simulink model "Csm_HighLvlArchitecture"  (R2017b)
settings: Solver=VariableStepAuto  StartTime=0.0  StopTime=10.0  RelTol=1e-3
undefined symbols (not defined in the file): accEgoVeh, Acceleration, apsEgoVeh, bpEgoVeh, Coasting, Control, CurrentDrivingLane, Curvature, CutIn, CutOut, Decelleration, distEgo2TS, distPredVeh, EgoVeh_State, EgoVehicle, GRG, Idle, ITS, Localization, Management, MATLAB, Mobileye, Obstacles, Obstacles_State, Perception, posEgoVeh, posGear, posTrafficSignal, PrecedingVehicle, Prediction, Python, Regen, Run, Slope, spdEgoVeh, spdMot, spdPredVeh, SpeedLimit, SRG, Stop, Topography, Topography_State, trqMot, Type, user_define_author, user_define_category, user_define_platform, Visual_C, yawEgoVeh
libraries: DX_Lib x1
(part 2 of 2)

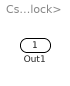
== system Csm_HighLvlArchitecture/<ArchitectureBlock> ==
  Out1 : Outport

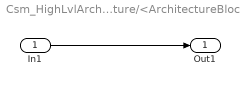
== system Csm_HighLvlArchitecture/<ArchitectureBlock>1 ==
  In1 : Inport
  Out1 : Outport
  wires:
  In1/1 -> Out1/1

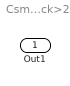
== system Csm_HighLvlArchitecture/<ArchitectureBlock>2 ==
  Out1 : Outport

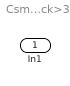
== system Csm_HighLvlArchitecture/<ArchitectureBlock>3 ==
  In1 : Inport

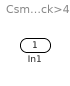
== system Csm_HighLvlArchitecture/<ArchitectureBlock>4 ==
  In1 : Inport

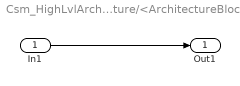
== system Csm_HighLvlArchitecture/<ArchitectureBlock>5 ==
  In1 : Inport
  Out1 : Outport
  wires:
  In1/1 -> Out1/1

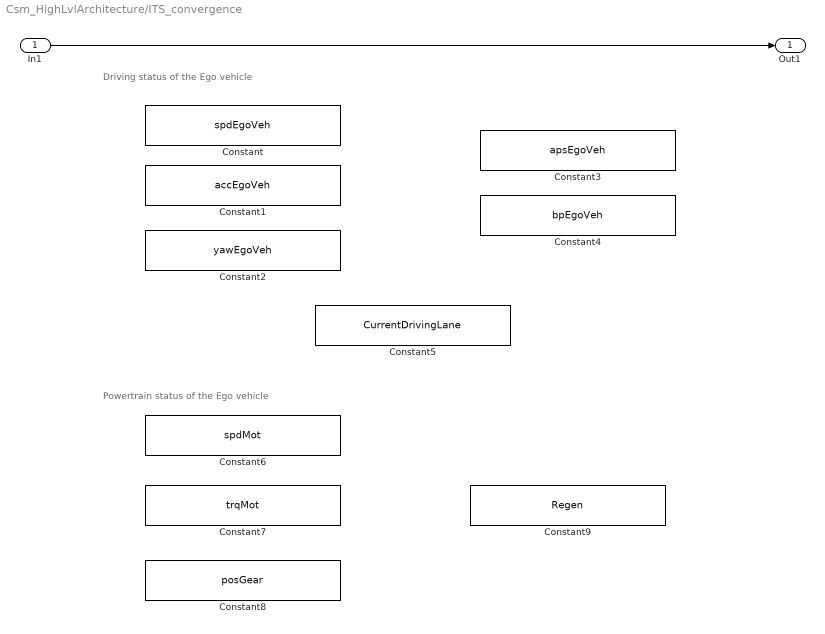
== system Csm_HighLvlArchitecture/ITS_convergence  ==
  note: Powertrain status of the Ego vehicle
  note: Driving status of the Ego vehicle
  In1 : Inport
  Constant : Constant  Value=spdEgoVeh
  Constant1 : Constant  Value=accEgoVeh
  Constant2 : Constant  Value=yawEgoVeh
  Constant3 : Constant  Value=apsEgoVeh
  Constant4 : Constant  Value=bpEgoVeh
  Constant5 : Constant  Value=CurrentDrivingLane
  Constant6 : Constant  Value=spdMot
  Constant7 : Constant  Value=trqMot
  Constant8 : Constant  Value=posGear
  Constant9 : Constant  Value=Regen
  Out1 : Outport
  wires:
  In1/1 -> Out1/1

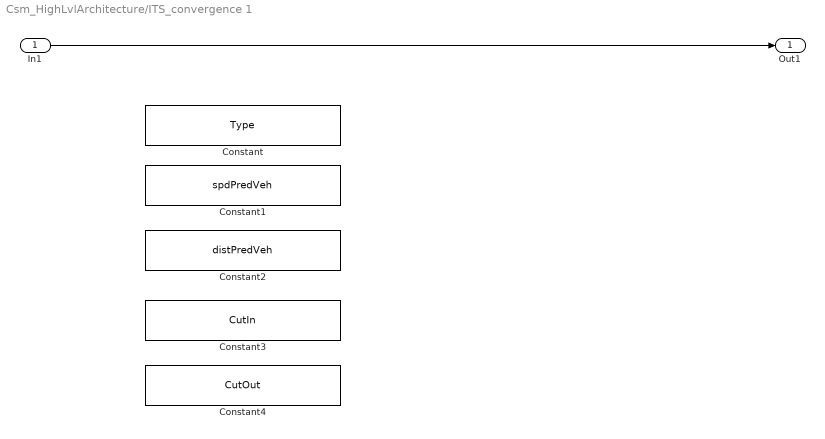
== system Csm_HighLvlArchitecture/ITS_convergence 1 ==
  In1 : Inport
  Constant : Constant  Value=Type
  Constant1 : Constant  Value=spdPredVeh
  Constant2 : Constant  Value=distPredVeh
  Constant3 : Constant  Value=CutIn
  Constant4 : Constant  Value=CutOut
  Out1 : Outport
  wires:
  In1/1 -> Out1/1

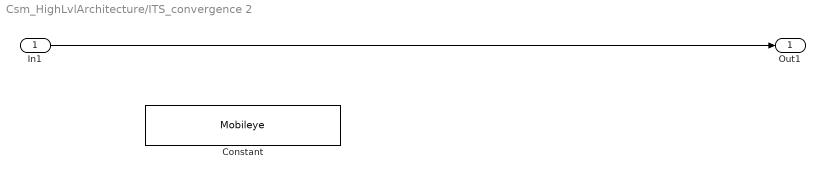
== system Csm_HighLvlArchitecture/ITS_convergence 2 ==
  In1 : Inport
  Constant : Constant  Value=Mobileye
  Out1 : Outport
  wires:
  In1/1 -> Out1/1

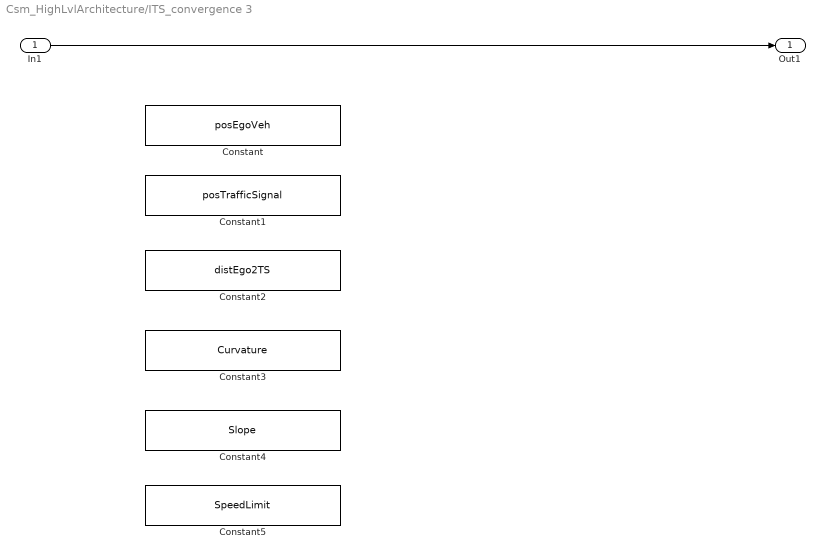
== system Csm_HighLvlArchitecture/ITS_convergence 3 ==
  In1 : Inport
  Constant : Constant  Value=posEgoVeh
  Constant1 : Constant  Value=posTrafficSignal
  Constant2 : Constant  Value=distEgo2TS
  Constant3 : Constant  Value=Curvature
  Constant4 : Constant  Value=Slope
  Constant5 : Constant  Value=SpeedLimit
  Out1 : Outport
  wires:
  In1/1 -> Out1/1

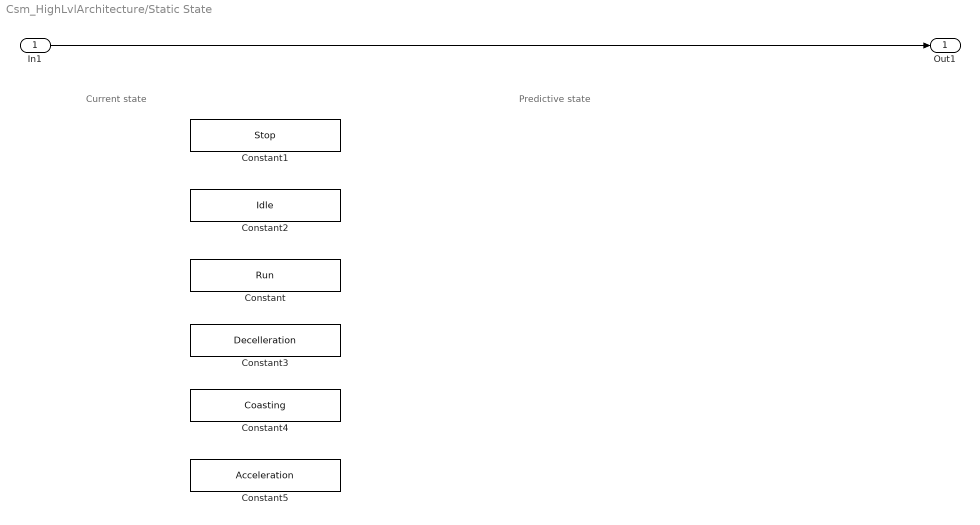
== system Csm_HighLvlArchitecture/Static State  ==
  note: Predictive state
  note: Current state
  In1 : Inport
  Constant : Constant  Value=Run
  Constant1 : Constant  Value=Stop
  Constant2 : Constant  Value=Idle
  Constant3 : Constant  Value=Decelleration
  Constant4 : Constant  Value=Coasting
  Constant5 : Constant  Value=Acceleration
  Out1 : Outport
  wires:
  In1/1 -> Out1/1
